simulink model "course_loop"  (R2016a)
settings: Solver=VariableStepAuto  StartTime=0.0  StopTime=20  RelTol=1e-3
values from neighbouring files (symbols this model uses):
  course_ki = wn_course^2 * 10 / 9.81    (= 0.229243394371)    [tune_course.m]
  course_kp = 2*zeta_course * wn_course * 10 / 9.81    (= 4.83408086986)    [tune_course.m]
settings Model: Creator=andreanv  LastModifiedBy=andreanv

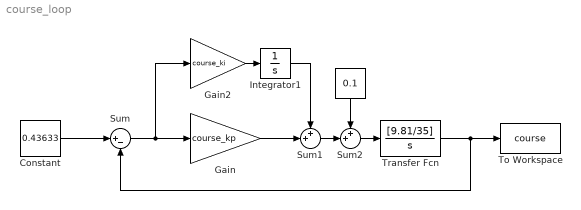
== system course_loop ==
  " " : Constant  Value=0.1
  Constant : Constant  Value=0.43633
  Gain : Gain  Gain=course_kp
  Gain2 : Gain  Gain=course_ki
  Integrator1 : Integrator
  Sum : Sum  Inputs=|+-
  Sum1 : Sum  Inputs=++|
  Sum2 : Sum  Inputs=++|
  To Workspace : ToWorkspace  VariableName=course  SaveFormat=Timeseries  SampleTime=-1
  Transfer Fcn : TransferFcn  Numerator=[9.81/35]  Denominator=[1 0]
  wires:
  Constant/1 -> Sum/1
  Sum/1 -> Gain2/1, Gain/1
  Sum1/1 -> Sum2/2
  Sum2/1 -> Transfer Fcn/1
  " "/1 -> Sum2/1
  Gain2/1 -> Integrator1/1
  Integrator1/1 -> Sum1/1
  Gain/1 -> Sum1/2
  Transfer Fcn/1 -> Sum/2, To Workspace/1
